simulink model "F16ASYM_Controlled_ACC"  (R2012b)
settings: Solver=ode3  SolverMode=SingleTasking  StartTime=0.0  StopTime=inf  FixedStep=T_sim  RelTol=1e-3
InitFcn:
  | load('NN_c_weights_Last_stable.mat')
values from neighbouring files (symbols this model uses):
  a1 = fitresult.p1    [Stall_protection.m]
  alpha_map_eval = ones(size(M_eval))*NaN    [Auto_trim_aid.m]    (also in Autotrim_maps.mat = [nan nan 0.277598136245 0.119432432992 0.0579479097061 0.027)
  beta_map_eval = ones(size(M_eval))*NaN    [Auto_trim_aid.m]    (also in Autotrim_maps.mat = [nan nan -0.00151549403324 0.00117807579006 -0.0052086799721)
  C_L_0 = fitresult.p2    [Stall_protection.m]
  G_eval = NaN*ones(size(M_sq,2),size(H_sq,2))    [Stall_protection.m]
  H_sq = unique(sort(H_sq))    [Stall_protection.m]
  H_sq_autotrim = min( F_envelope.H_1g):2000:max(F_envelope.H_1g)    [Auto_trim_aid.m]    (also in Autotrim_maps.mat = [0 2000 4000 6000 8000 10000 12000 14000 16000 18000])
  K_b_ACC = params(3)    [Cost_function.m]
  K_b_q = params(4)    [Cost_function.m]
  learning = 20    [Scheduling_desing.m]
  M_sq = unique(sort(M_sq))    [Stall_protection.m]
  M_sq_autotrim = 0:0.1:max(F_envelope.M_1g)    [Auto_trim_aid.m]    (also in Autotrim_maps.mat = [0 0.1 0.2 0.3 0.4 0.5 0.6 0.7 0.8 0.9 1 1.1 ... (21 element)
  Model_used_flag = 1    [Scheduling_desing.m]
  reg_param = 1    [Scheduling_desing.m]
  T_sim = 0.04    [Run_me.m]    (also in Scheduling_desing.m = 0.02)
  tau_ACC = params(1)    [Cost_function.m]
  tau_q = params(2)    [Cost_function.m]
  V_Comp_A_w_z_last = [-0.043311742939 0.0085685727899 -0.0213735657625 0.0330213821126 -0.0306555996667 -0.00573122365227 -0.0106441480787 0.0329440631876 0.0177121952361 -0.0290685435098 -0.0181457235686 -0.0361990502411 ... (1250 elements, 50x25)]    [NN_c_weights_Last_stable.mat]
  V_Comp_last = [-0.0421958473648 0.0184516098779 -0.0436695953504 -0.041154016657 0.00216882652165 -0.0388561228631 0.0327521861474 0.0326079628857 0.0227071838361 -0.0338588476214 0.0161615063846 0.00186003522421 ... (1250 elements, 50x25)]    [NN_c_weights_Last_stable.mat]
  velocity = M_eval(I,J)*a    [Auto_trim_aid.m]    (also in Scheduling_desing.m = M_eval_sche(I,J)*a)
  W_Comp_A_w_z_last = [-0.00689921461652 0.00234704735165 -0.000126421245896 0.00121944724496 6.17702028018e-05 -0.000422762754226 -0.000228913732743 -1.1618795843e-05 7.94007436465e-05 0.000588815786054 2.98617078429e-05 -0.00020420127191 ... (153 elements, 3x51)]    [NN_c_weights_Last_stable.mat]
  W_Comp_last = [-0.00864477030284 0.000183920433695 -0.000300268209456 0.00178165628538 -0.000144806488148 -0.000715209966 -0.000733452792184 5.9552378004e-05 0.000293789747621 0.00184648331608 -0.000150090451416 -0.000741280397229 ... (153 elements, 3x51)]    [NN_c_weights_Last_stable.mat]
undefined symbols (not defined in the file or in its folder): B, DiscIntNeverNeededParam, fi_flag_Simulink, k_B, m_B, sigbuilder_block, Stall_curve, Theta_1_roll_last, Theta_2_roll_last, Theta_3_roll_last, trim_control, trim_state, trim_throttle, V_long_lastA_w_z, V_long_lastAoA, V_roll_last, V_roll_lastMOD, V_yaw_last, W_long_lastA_w_z, W_long_lastAoA, W_roll_last, W_roll_lastMOD, W_yaw_last
libraries: Adaptive_FaultTolerantControl x43, F16_Actuator_Library x14, dspsigops x13, simulink x8, dsparch4 x6, simulink_extras x5, aerolibatmos2 x5, aerolibtransform2 x5, dspmtrx3 x3, qcatlib x2, dspvision x2, dspsnks4 x2
(part 7 of 10)

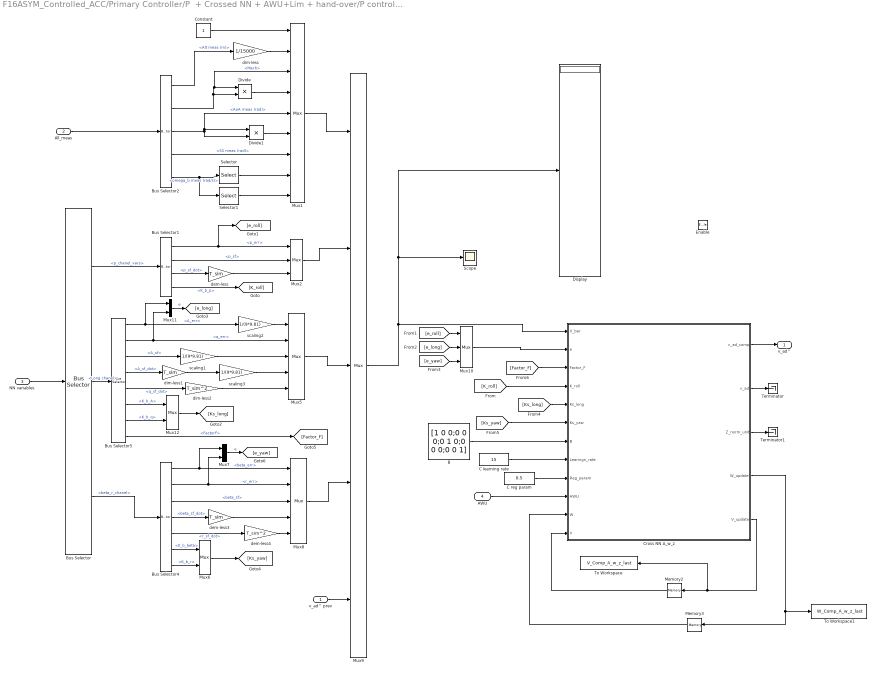
== system F16ASYM_Controlled_ACC/Primary Controller/P  + Crossed NN + AWU+Lim + hand-over/P controller + adaptive Crossed NN + AWU+Lim    in ACC /Complete crossed On-line (adaptive) multi-layer NN: A_w_z ==
  v_ad^ prev : Inport
  All_meas : Inport  Port=2
  NN variables : Inport  Port=3
  AWU : Inport  Port=4
  Enable : EnablePort  StatesWhenEnabling=reset
  B : Constant  Value=[1 0 0;0 0 0;0 1 0;0 0 0;0 0 1]
  Bus Selector : BusSelector  OutputSignals=p_chanel_vars,Long chanel,beta_r_chanel
  Bus Selector1 : BusSelector  OutputSignals=p_err,p_sf,p_sf_dot,K_b_p
  Bus Selector2 : BusSelector  OutputSignals=signal1.Alt meas (m),signal2.Mach,signal1.AoA meas (rad),signal1.SS meas (rad),signal1.omega_b meas (rad/s)
  Bus Selector4 : BusSelector  OutputSignals=beta_chanel vars.beta_err,r_chanel vars.r_err,beta_chanel vars.beta_sf,beta_chanel vars.beta_sf_dot,r_chanel vars.r_sf_dot,beta_chanel vars.K_b_beta,r_chanel vars.K_b_r
  Bus Selector5 : BusSelector  OutputSignals=A_chanel vars.A_err,q_chanel_vars.q_err,A_chanel vars.A_sf,A_chanel vars.A_sf_dot,q_chanel_vars.q_sf_dot,A_chanel vars.K_b_A,q_chanel_vars.K_b_q,A_chanel vars.FactorF
  C learning rate : Constant  Value=15  SampleTime=T_sim
  C reg param : Constant  Value=0.5  SampleTime=T_sim
  Constant : Constant
  Cross NN A_w_z : MATLAB Function  TreatAsAtomicUnit=on
  Display : Display
  Divide : Product  Inputs=**
  Divide1 : Product  Inputs=**
  Memory2 : Memory  X0=V_Comp_A_w_z_last
  Memory3 : Memory  X0=W_Comp_A_w_z_last
  Mux1 : Mux  Inputs=9
  Mux10 : Mux  Inputs=3
  Mux{6..7,11..12} (4 alike) : Mux  Inputs=2
  Mux2 : Mux  Inputs=3
  Mux5 : Mux  Inputs=5
  Mux8 : Mux  Inputs=5
  Mux9 : Mux  Inputs=[9 3 5 5 3]
  Scope : Scope
      settings: SaveName=ScopeData8
  Selector : Selector  InputPortWidth=3  IndexOptions=Index vector (dialog)  Indices=1  OutputSizes=1
  Selector1 : Selector  InputPortWidth=3  IndexOptions=Index vector (dialog)  Indices=3  OutputSizes=1
  Terminator : Terminator
  Terminator1 : Terminator
  To Workspace : ToWorkspace  VariableName=V_Comp_A_w_z_last  SampleTime=-1
      settings: MaxDataPoints=1
  To Workspace1 : ToWorkspace  VariableName=W_Comp_A_w_z_last  SampleTime=-1
      settings: MaxDataPoints=1
  dem-less : Gain  Gain=T_sim
  dem-less3 : Gain  Gain=T_sim
  dem-less4 : Gain  Gain=T_sim^2
  dim-less : Gain  Gain=1/15000
  dim-less1 : Gain  Gain=T_sim
  dim-less2 : Gain  Gain=T_sim^2
  scaling1 : Gain  Gain=1/(9*9.81)
  scaling2 : Gain  Gain=1/(9*9.81)
  scaling3 : Gain  Gain=1/(9*9.81)
  v_ad^ : Outport
  wires:
  [Factor_F] -> Cross NN A_w_z/3(Factor_F)
  Bus Selector5/8 -> [Factor_F]  "<FactorF>"
  scaling3/1 -> Mux5/4
  dim-less2/1 -> Mux5/5
  scaling1/1 -> Mux5/3
  Mux11/1 -> [e_long]  "e"
  Bus Selector/2 -> Bus Selector5/1  "<Long chanel>"
  Bus Selector5/1 -> Mux11/1, scaling2/1  "<A_err>"
  Bus Selector5/2 -> Mux11/2, Mux5/2  "<q_err>"
  Bus Selector5/3 -> scaling1/1  "<A_sf>"
  Bus Selector5/4 -> dim-less1/1  "<A_sf_dot>"
  Bus Selector5/5 -> dim-less2/1  "<q_sf_dot>"
  Bus Selector5/7 -> Mux12/2  "<K_b_q>"
  Bus Selector5/6 -> Mux12/1  "<K_b_A>"
  scaling2/1 -> Mux5/1
  dim-less1/1 -> scaling3/1
  Selector1/1 -> Mux1/9
  [Ks_yaw] -> Cross NN A_w_z/6(Ks_yaw)
  [Ks_long] -> Cross NN A_w_z/5(Ks_long)
  [K_roll] -> Cross NN A_w_z/4(K_roll)
  [e_yaw] -> Mux10/3
  [e_long] -> Mux10/2
  [e_roll] -> Mux10/1
  Mux10/1 -> Cross NN A_w_z/2(e)
  Cross NN A_w_z/4(W_update) -> To Workspace1/1, Memory3/1
  Cross NN A_w_z/5(V_update) -> Memory2/1, To Workspace/1
  Cross NN A_w_z/2(v_ad) -> Terminator/1
  B/1 -> Cross NN A_w_z/7(B)
  Memory3/1 -> Cross NN A_w_z/11(W)
  Memory2/1 -> Cross NN A_w_z/12(V)
  Cross NN A_w_z/1(v_ad_comp) -> v_ad^/1
  C learning rate/1 -> Cross NN A_w_z/8(Learnign_rate)
  C reg param/1 -> Cross NN A_w_z/9(Reg_param)
  Cross NN A_w_z/3(Z_norm_unit) -> Terminator1/1
  Mux9/1 -> Cross NN A_w_z/1(X_bar), Display/1, Scope/1
  v_ad^ prev/1 -> Mux9/5
  Mux8/1 -> Mux9/4
  Mux5/1 -> Mux9/3
  Mux2/1 -> Mux9/2
  Mux1/1 -> Mux9/1
  dem-less4/1 -> Mux8/5
  Mux7/1 -> [e_yaw]  "e"
  Bus Selector4/2 -> Mux7/2, Mux8/2  "<r_err>"
  Bus Selector4/1 -> Mux7/1, Mux8/1  "<beta_err>"
  Mux6/1 -> [Ks_yaw]
  Bus Selector4/6 -> Mux6/1  "<K_b_beta>"
  Bus Selector4/7 -> Mux6/2  "<K_b_r>"
  Bus Selector4/5 -> dem-less4/1  "<r_sf_dot>"
  Bus Selector4/4 -> dem-less3/1  "<beta_sf_dot>"
  Bus Selector4/3 -> Mux8/3  "<beta_sf>"
  dem-less3/1 -> Mux8/4
  Mux12/1 -> [Ks_long]
  dem-less/1 -> Mux2/3
  Bus Selector1/1 -> Mux2/1, [e_roll]  "<p_err>"
  Bus Selector1/2 -> Mux2/2  "<p_sf>"
  Bus Selector1/4 -> [K_roll]  "<K_b_p>"
  Bus Selector2/3 -> Divide1/2, Mux1/5, Divide1/1  "<AoA meas (rad)>"
  Bus Selector2/2 -> Divide/1, Mux1/3, Divide/2  "<Mach>"
  Bus Selector2/4 -> Mux1/7  "<SS meas (rad)>"
  Selector/1 -> Mux1/8
  Bus Selector1/3 -> dem-less/1  "<p_sf_dot>"
  Constant/1 -> Mux1/1
  All_meas/1 -> Bus Selector2/1
  Bus Selector2/1 -> dim-less/1  "<Alt meas (m)>"
  Divide/1 -> Mux1/4
  Divide1/1 -> Mux1/6
  dim-less/1 -> Mux1/2
  Bus Selector2/5 -> Selector/1, Selector1/1  "<omega_b meas (rad/s)>"
  NN variables/1 -> Bus Selector/1
  Bus Selector/1 -> Bus Selector1/1  "<p_chanel_vars>"
  Bus Selector/3 -> Bus Selector4/1  "<beta_r_chanel>"
  AWU/1 -> Cross NN A_w_z/10(AWU)

== system F16ASYM_Controlled_ACC/Primary Controller/P  + Crossed NN + AWU+Lim + hand-over/P controller + adaptive Crossed NN + AWU+Lim    in ACC /Lat_dir Dyn Inversion: beta_dot->r_c ==
  beta_dot_c : Inport
  All_meas : Inport  Port=2
  A_w_y : Selector  InputPortWidth=3  IndexOptions=Index vector (dialog)  Indices=2  OutputSizes=1
  Bus Selector : BusSelector  OutputSignals=signal1.AoA meas (rad),signal1.omega_b meas (rad/s),signal1.V_TAS (m/s),signal2.A_w_CG
  Divide1 : Product  Inputs=**
  Divide3 : Product  Inputs=**
  Divide4 : Product  Inputs=/*
  Divide5 : Product  Inputs=*/
  Selector : Selector  InputPortWidth=3  IndexOptions=Index vector (dialog)  Indices=1  OutputSizes=1
  Trigonometric Function : Trigonometry  Operator=cos
  Trigonometric Function3 : Trigonometry  Operator=tan
  "q_c " : Sum  Inputs=-++
  r_c : Outport
  wires:
  "q_c "/1 -> r_c/1
  Bus Selector/1 -> Trigonometric Function/1, Trigonometric Function3/1  "<AoA meas (rad)>"
  Bus Selector/2 -> Selector/1  "<omega_b meas (rad/s)>"
  Divide1/1 -> "q_c "/2
  Divide3/1 -> Divide4/1
  A_w_y/1 -> Divide4/2
  All_meas/1 -> Bus Selector/1
  Bus Selector/4 -> A_w_y/1  "<A_w_CG>"
  Divide4/1 -> "q_c "/3
  Bus Selector/3 -> Divide3/2  "<V_TAS (m/s)>"
  Trigonometric Function/1 -> Divide3/1, Divide5/2
  Divide5/1 -> "q_c "/1
  beta_dot_c/1 -> Divide5/1
  Trigonometric Function3/1 -> Divide1/1
  Selector/1 -> Divide1/2

== system F16ASYM_Controlled_ACC/Primary Controller/P  + Crossed NN + AWU+Lim + hand-over/P controller + adaptive Crossed NN + AWU+Lim    in ACC /Long Dyn Inversion: alpha_dot ->q ==
  alpha_dot_c : Inport
  All_meas : Inport  Port=2
  Completed : Subsystem
  Manual Switch : ManualSwitch
  Simplified : Subsystem
  q_c : Outport
  wires:
  alpha_dot_c/1 -> Simplified/1(alpha_dot_c), Completed/1(alpha_dot_c)
  All_meas/1 -> Simplified/2(All_meas), Completed/2(All_meas)
  Completed/1(q_c) -> Manual Switch/1
  Simplified/1(q_c) -> Manual Switch/2
  Manual Switch/1 -> q_c/1

== system F16ASYM_Controlled_ACC/Primary Controller/P  + Crossed NN + AWU+Lim + hand-over/P controller + adaptive Crossed NN + AWU+Lim    in ACC /Longitudinal controller in A_w_z ==
  A_w_z des : Inport
  AoA des (rad) : Inport  Port=2
  Anti-windup A_w_z : Inport  Port=3
  Anti-windup AoA : Inport  Port=4
  All meas : Inport  Port=5
  Accel rate --> AoA rate! : Subsystem
  Bus Creator : BusCreator  Inputs=5
  Bus Selector : BusSelector  OutputSignals=signal2.A_w_CG
  Divide : Product  Inputs=**
  Gain : Gain  Gain=-1
  Ref Model and P Controller : Adaptive_FaultTolerantControl/Ref Model and P Controller  tau=0.3  y_i=0  K_f=1  K_b=2.5
  Selector : Selector  InputPortWidth=3  IndexOptions=Index vector (dialog)  Indices=3  OutputSizes=1
  Stall protection : Subsystem  Commented=on
  Sum : Sum  Inputs=+-|
  Terminator : Terminator
  Terminator1 : Terminator
  Terminator2 : Terminator
  A_chanel vars : Outport
  alpha_dot_c : Outport  Port=2
  wires:
  Anti-windup AoA/1 -> Terminator1/1
  AoA des (rad)/1 -> Terminator/1
  Selector/1 -> Gain/1
  Gain/1 -> Ref Model and P Controller/2
  Bus Selector/1 -> Selector/1  "<A_w_CG>"
  Anti-windup A_w_z/1 -> Terminator2/1
  A_w_z des/1 -> Ref Model and P Controller/1
  Ref Model and P Controller/1 -> Divide/1
  Ref Model and P Controller/2 -> Bus Creator/1  "A_sf_dot"
  Ref Model and P Controller/3 -> Bus Creator/2, Sum/1  "A_sf"
  Sum/1 -> Bus Creator/3  "A_err"
  Ref Model and P Controller/4 -> Sum/2
  Ref Model and P Controller/5 -> Bus Creator/4  "K_b_A"
  Bus Creator/1 -> A_chanel vars/1
  Divide/1 -> alpha_dot_c/1
  Accel rate --> AoA rate!/1(A_w  to AoA rates factor) -> Bus Creator/5, Divide/2  "FactorF"
  All meas/1 -> Bus Selector/1, Stall protection/2(All meas), Accel rate --> AoA rate!/1(All_meas)

== system F16ASYM_Controlled_ACC/Primary Controller/P  + Crossed NN + AWU+Lim + hand-over/P controller + adaptive Crossed NN + AWU+Lim    in ACC /Physical limitation ==
  note: Converto to Angular accelerations
  v comm : Inport
  all meas : Inport  Port=2
  Ang Accel : MATLAB Function
  Bus Selector : BusSelector  OutputSignals=signal1.Alt meas (m),signal1.V_TAS (m/s),signal1.AoA meas (rad),signal1.SS meas (rad),signal1.omega_b meas (rad/s),signal1.Throttle_meas
  Bus Selector1 : BusSelector  OutputSignals=signal2.q (Pa),signal1.omega_b meas (rad/s)
  Demux : Demux  Outputs=3
  Display : Display
  Display1 : Display
  Display2 : Display
  Divide : Product  Inputs=**
  Divide1 : Product  Inputs=**
  Gain : Gain  Gain=-1
  Gain1 : Gain
  Mom coefficients that was reached : MATLABFcn  MATLABFcn=Moms_Coeff_estimator  OutputDimensions=3  OutputSignalType=real
  Moments : Subsystem
  Mux : Mux  Inputs=3
  Mux1 : Mux  Inputs=7
  Saturation Dynamic : simulink/Discontinuities/Saturation Dynamic  OutMin=[]  OutMax=[]  OutDataTypeStr=Inherit: Same as second input  OutDataType=fixdt(1, 16)  OutScaling=2^-10  DoSatur=off
  Sign : Signum
  Sign1 : Signum
  max deflections estimator : MATLAB Function  TreatAsAtomicUnit=on
  v limted : Outport
  wires:
  max deflections estimator/1(max_defl) -> Mux1/7
  Mux1/1 -> Mom coefficients that was reached/1
  Bus Selector/5 -> Mux1/5  "<omega_b meas (rad/s)>"
  Bus Selector/1 -> Mux1/1  "<Alt meas (m)>"
  Bus Selector/2 -> Mux1/2  "<V_TAS (m/s)>"
  Bus Selector/3 -> Mux1/3  "<AoA meas (rad)>"
  Bus Selector/4 -> Mux1/4  "<SS meas (rad)>"
  Bus Selector/6 -> Mux1/6  "<Throttle_meas>"
  Ang Accel/2(q_dot) -> Mux/2
  Ang Accel/3(r_dot) -> Mux/3
  Ang Accel/1(p_dot) -> Mux/1
  Bus Selector1/2 -> Ang Accel/4(omega_b)  "<omega_b meas (rad/s)>"
  Moments/3(N) -> Ang Accel/3(N)
  Moments/2(M) -> Ang Accel/2(M)
  Moments/1(L) -> Ang Accel/1(L)
  Bus Selector1/1 -> Moments/4(q)  "<q (Pa)>"
  Demux/3 -> Moments/3(C_N)
  Demux/2 -> Moments/2(C_M)
  Demux/1 -> Moments/1(C_L)
  Mom coefficients that was reached/1 -> Demux/1
  all meas/1 -> Bus Selector/1, Bus Selector1/1
  Mux/1 -> Gain1/1
  v comm/1 -> Saturation Dynamic/2, Display1/1, max deflections estimator/1(v_comm)
  Saturation Dynamic/1 -> Display/1, v limted/1
  Sign/1 -> Divide/1
  Gain1/1 -> Divide/2, Divide1/1, Sign1/1, Display2/1, Sign/1
  Sign1/1 -> Gain/1
  Divide/1 -> Saturation Dynamic/1
  Gain/1 -> Divide1/2
  Divide1/1 -> Saturation Dynamic/3

== system F16ASYM_Controlled_ACC/Primary Controller/P  + Crossed NN + AWU+Lim + hand-over/P controller + adaptive Crossed NN + AWU+Lim    in ACC /Sigmoid  ==
  In : Inport
  Display : Display
  Fcn1 : Fcn  Commented=on  Expr=2.0 ./ (1.0 + exp(-u(4)*u(1:3)))-1
  MATLAB Function : MATLAB Function  TreatAsAtomicUnit=on
  a : Constant  Value=a
  Out : Outport
  wires:
  MATLAB Function/1(y) -> Display/1, Out/1
  In/1 -> MATLAB Function/1(u)
  a/1 -> MATLAB Function/2(a)

== system F16ASYM_Controlled_ACC/Primary Controller/P  + Crossed NN + AWU+Lim + hand-over/P controller + adaptive Crossed NN + AWU+Lim   in AoA/Body Rates Controller ==
  p_ref : Inport
  q_ref : Inport  Port=2
  r_ref : Inport  Port=3
  All_meas : Inport  Port=4
  Bus Creator : BusCreator
  Bus Creator1 : BusCreator
  Bus Creator2 : BusCreator
  Bus Selector : BusSelector  OutputSignals=signal1.omega_b meas (rad/s)
  Display1 : Display
  Mux : Mux  Inputs=3
  Ref Model and P Controller p : Adaptive_FaultTolerantControl/Ref Model and P Controller  tau=0.1  y_i=trim_state(10)  K_f=1  K_b=7
  Ref Model and P Controller q : Adaptive_FaultTolerantControl/Ref Model and P Controller  tau=0.06  y_i=trim_state(11)  K_f=1  K_b=1
  Ref Model and P Controller r : Adaptive_FaultTolerantControl/Ref Model and P Controller  tau=0.2  y_i=trim_state(12)  K_f=1  K_b=4
  Selector : Selector  InputPortWidth=3  IndexOptions=Index vector (dialog)  Indices=1  OutputSizes=1
  Selector1 : Selector  InputPortWidth=3  IndexOptions=Index vector (dialog)  Indices=2  OutputSizes=1
  Selector2 : Selector  InputPortWidth=3  IndexOptions=Index vector (dialog)  Indices=3  OutputSizes=1
  Sum : Sum  Inputs=+-|
  Sum1 : Sum  Inputs=+-|
  Sum2 : Sum  Inputs=+-|
  q_chanel vars : Outport
  p_chanel vars : Outport  Port=2
  r_chanel vars : Outport  Port=3
  Angular acc des (rad/s^2) : Outport  Port=4
  wires:
  All_meas/1 -> Bus Selector/1
  Bus Selector/1 -> Selector/1, Selector1/1, Selector2/1  "<omega_b meas (rad/s)>"
  p_ref/1 -> Ref Model and P Controller p/1
  Selector/1 -> Ref Model and P Controller p/2
  Ref Model and P Controller p/1 -> Mux/1
  Mux/1 -> Angular acc des (rad/s^2)/1
  q_ref/1 -> Ref Model and P Controller q/1
  Selector1/1 -> Ref Model and P Controller q/2
  r_ref/1 -> Ref Model and P Controller r/1
  Ref Model and P Controller q/1 -> Mux/2
  Ref Model and P Controller r/1 -> Mux/3
  Ref Model and P Controller p/2 -> Bus Creator/1  "p_sf_dot"
  Ref Model and P Controller p/3 -> Sum/1, Bus Creator/2  "p_sf"
  Sum/1 -> Display1/1, Bus Creator/3  "p_err"
  Bus Creator/1 -> p_chanel vars/1
  Bus Creator1/1 -> q_chanel vars/1
  Bus Creator2/1 -> r_chanel vars/1
  Selector2/1 -> Ref Model and P Controller r/2
  Ref Model and P Controller p/4 -> Sum/2
  Ref Model and P Controller p/5 -> Bus Creator/4  "K_b_p"
  Ref Model and P Controller q/2 -> Bus Creator1/1  "q_sf_dot"
  Ref Model and P Controller q/3 -> Sum1/1, Bus Creator1/2  "q_sf"
  Sum1/1 -> Bus Creator1/3  "q_err"
  Ref Model and P Controller q/4 -> Sum1/2
  Ref Model and P Controller q/5 -> Bus Creator1/4  "K_b_q"
  Ref Model and P Controller r/2 -> Bus Creator2/1  "r_sf_dot"
  Ref Model and P Controller r/3 -> Sum2/1, Bus Creator2/2  "r_sf"
  Sum2/1 -> Bus Creator2/3  "r_err"
  Ref Model and P Controller r/4 -> Sum2/2
  Ref Model and P Controller r/5 -> Bus Creator2/4  "K_b_r"

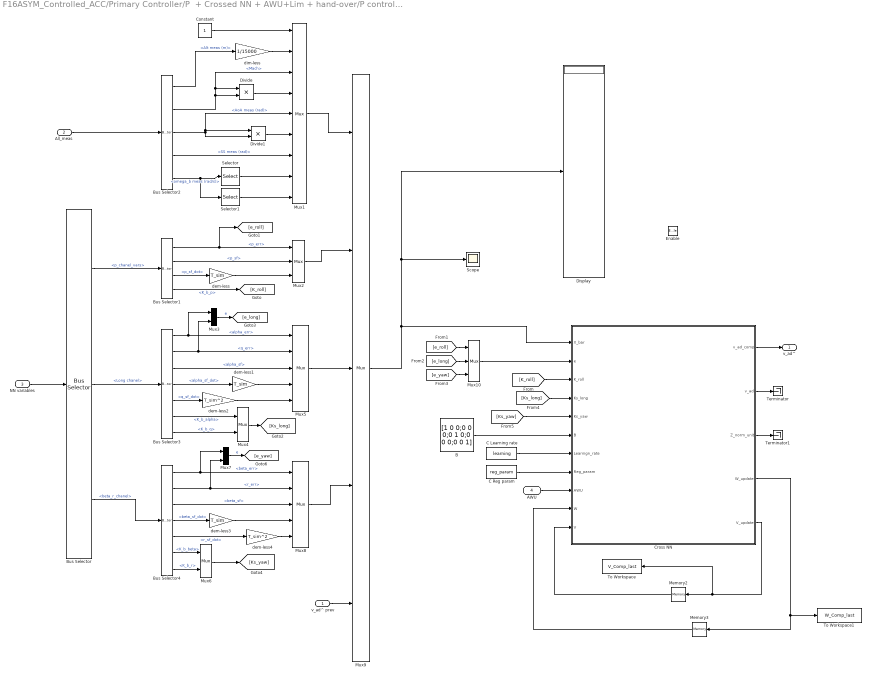
== system F16ASYM_Controlled_ACC/Primary Controller/P  + Crossed NN + AWU+Lim + hand-over/P controller + adaptive Crossed NN + AWU+Lim   in AoA/Complete crossed On-line (adaptive) multi-layer NN: AoA ==
  v_ad^ prev : Inport
  All_meas : Inport  Port=2
  NN variables : Inport  Port=3
  AWU : Inport  Port=4
  Enable : EnablePort  StatesWhenEnabling=reset
  B : Constant  Value=[1 0 0;0 0 0;0 1 0;0 0 0;0 0 1]
  Bus Selector : BusSelector  OutputSignals=p_chanel_vars,Long chanel,beta_r_chanel
  Bus Selector1 : BusSelector  OutputSignals=p_err,p_sf,p_sf_dot,K_b_p
  Bus Selector2 : BusSelector  OutputSignals=signal1.Alt meas (m),signal2.Mach,signal1.AoA meas (rad),signal1.SS meas (rad),signal1.omega_b meas (rad/s)
  Bus Selector3 : BusSelector  OutputSignals=alpha_chanel vars.alpha_err,q_chanel_vars.q_err,alpha_chanel vars.alpha_sf,alpha_chanel vars.alpha_sf_dot,q_chanel_vars.q_sf_dot,alpha_chanel vars.K_b_alpha,q_chanel_vars.K_b_q
  Bus Selector4 : BusSelector  OutputSignals=beta_chanel vars.beta_err,r_chanel vars.r_err,beta_chanel vars.beta_sf,beta_chanel vars.beta_sf_dot,r_chanel vars.r_sf_dot,beta_chanel vars.K_b_beta,r_chanel vars.K_b_r
  C Learning rate : Constant  Value=learning  SampleTime=T_sim
  C Reg param : Constant  Value=reg_param  SampleTime=T_sim
  Constant : Constant
  Cross NN : MATLAB Function  TreatAsAtomicUnit=on
  Display : Display
  Divide : Product  Inputs=**
  Divide1 : Product  Inputs=**
  Memory2 : Memory  X0=V_Comp_last
  Memory3 : Memory  X0=W_Comp_last
  Mux1 : Mux  Inputs=9
  Mux10 : Mux  Inputs=3
  Mux2 : Mux  Inputs=3
  Mux{3..4,6..7} (4 alike) : Mux  Inputs=2
  Mux5 : Mux  Inputs=5
  Mux8 : Mux  Inputs=5
  Mux9 : Mux  Inputs=[9 3 5 5 3]
  Scope : Scope
      settings: SaveName=ScopeData8
  Selector : Selector  InputPortWidth=3  IndexOptions=Index vector (dialog)  Indices=1  OutputSizes=1
  Selector1 : Selector  InputPortWidth=3  IndexOptions=Index vector (dialog)  Indices=3  OutputSizes=1
  Terminator : Terminator
  Terminator1 : Terminator
  To Workspace : ToWorkspace  VariableName=V_Comp_last  SampleTime=-1
      settings: MaxDataPoints=1
  To Workspace1 : ToWorkspace  VariableName=W_Comp_last  SampleTime=-1
      settings: MaxDataPoints=1
  dem-less : Gain  Gain=T_sim
  dem-less1 : Gain  Gain=T_sim
  dem-less2 : Gain  Gain=T_sim^2
  dem-less3 : Gain  Gain=T_sim
  dem-less4 : Gain  Gain=T_sim^2
  dim-less : Gain  Gain=1/15000
  v_ad^ : Outport
  wires:
  Bus Selector/3 -> Bus Selector4/1  "<beta_r_chanel>"
  Bus Selector/2 -> Bus Selector3/1  "<Long chanel>"
  Bus Selector/1 -> Bus Selector1/1  "<p_chanel_vars>"
  NN variables/1 -> Bus Selector/1
  Bus Selector2/5 -> Selector1/1, Selector/1  "<omega_b meas (rad/s)>"
  dim-less/1 -> Mux1/2
  Divide1/1 -> Mux1/6
  Divide/1 -> Mux1/4
  Bus Selector2/1 -> dim-less/1  "<Alt meas (m)>"
  All_meas/1 -> Bus Selector2/1
  Constant/1 -> Mux1/1
  Bus Selector1/3 -> dem-less/1  "<p_sf_dot>"
  Selector/1 -> Mux1/8
  Bus Selector2/4 -> Mux1/7  "<SS meas (rad)>"
  Bus Selector2/2 -> Divide/2, Mux1/3, Divide/1  "<Mach>"
  Bus Selector2/3 -> Divide1/1, Mux1/5, Divide1/2  "<AoA meas (rad)>"
  Bus Selector1/4 -> [K_roll]  "<K_b_p>"
  Bus Selector1/2 -> Mux2/2  "<p_sf>"
  Bus Selector1/1 -> [e_roll], Mux2/1  "<p_err>"
  dem-less/1 -> Mux2/3
  dem-less2/1 -> Mux5/5
  dem-less1/1 -> Mux5/4
  Mux4/1 -> [Ks_long]
  Bus Selector3/6 -> Mux4/1  "<K_b_alpha>"
  Bus Selector3/7 -> Mux4/2  "<K_b_q>"
  Bus Selector3/5 -> dem-less2/1  "<q_sf_dot>"
  Bus Selector3/4 -> dem-less1/1  "<alpha_sf_dot>"
  Bus Selector3/1 -> Mux5/1, Mux3/1  "<alpha_err>"
  Bus Selector3/2 -> Mux5/2, Mux3/2  "<q_err>"
  Bus Selector3/3 -> Mux5/3  "<alpha_sf>"
  Mux3/1 -> [e_long]  "e"
  dem-less3/1 -> Mux8/4
  Bus Selector4/3 -> Mux8/3  "<beta_sf>"
  Bus Selector4/4 -> dem-less3/1  "<beta_sf_dot>"
  Bus Selector4/5 -> dem-less4/1  "<r_sf_dot>"
  Bus Selector4/7 -> Mux6/2  "<K_b_r>"
  Bus Selector4/6 -> Mux6/1  "<K_b_beta>"
  Mux6/1 -> [Ks_yaw]
  Bus Selector4/1 -> Mux8/1, Mux7/1  "<beta_err>"
  Bus Selector4/2 -> Mux8/2, Mux7/2  "<r_err>"
  Mux7/1 -> [e_yaw]  "e"
  dem-less4/1 -> Mux8/5
  Mux1/1 -> Mux9/1
  Mux2/1 -> Mux9/2
  Mux5/1 -> Mux9/3
  Mux8/1 -> Mux9/4
  v_ad^ prev/1 -> Mux9/5
  Mux9/1 -> Scope/1, Display/1, Cross NN/1(X_bar)
  Cross NN/3(Z_norm_unit) -> Terminator1/1
  C Reg param/1 -> Cross NN/8(Reg_param)
  C Learning rate/1 -> Cross NN/7(Learnign_rate)
  Cross NN/1(v_ad_comp) -> v_ad^/1
  Memory2/1 -> Cross NN/11(V)
  Memory3/1 -> Cross NN/10(W)
  B/1 -> Cross NN/6(B)
  Cross NN/2(v_ad) -> Terminator/1
  Cross NN/5(V_update) -> To Workspace/1, Memory2/1
  Cross NN/4(W_update) -> Memory3/1, To Workspace1/1
  Mux10/1 -> Cross NN/2(e)
  [e_roll] -> Mux10/1
  [e_long] -> Mux10/2
  [e_yaw] -> Mux10/3
  [K_roll] -> Cross NN/3(K_roll)
  [Ks_long] -> Cross NN/4(Ks_long)
  [Ks_yaw] -> Cross NN/5(Ks_yaw)
  Selector1/1 -> Mux1/9
  AWU/1 -> Cross NN/9(AWU)

== system F16ASYM_Controlled_ACC/Primary Controller/P  + Crossed NN + AWU+Lim + hand-over/P controller + adaptive Crossed NN + AWU+Lim   in AoA/Lat_dir Dyn Inversion: beta_dot->r_c ==
  beta_dot_c : Inport
  All_meas : Inport  Port=2
  A_w_y : Selector  InputPortWidth=3  IndexOptions=Index vector (dialog)  Indices=2  OutputSizes=1
  Bus Selector : BusSelector  OutputSignals=signal1.AoA meas (rad),signal1.omega_b meas (rad/s),signal1.V_TAS (m/s),signal2.A_w_CG
  Divide1 : Product  Inputs=**
  Divide3 : Product  Inputs=**
  Divide4 : Product  Inputs=/*
  Divide5 : Product  Inputs=*/
  Selector : Selector  InputPortWidth=3  IndexOptions=Index vector (dialog)  Indices=1  OutputSizes=1
  Trigonometric Function : Trigonometry  Operator=cos
  Trigonometric Function3 : Trigonometry  Operator=tan
  "q_c " : Sum  Inputs=-++
  r_c : Outport
  wires:
  "q_c "/1 -> r_c/1
  Bus Selector/1 -> Trigonometric Function/1, Trigonometric Function3/1  "<AoA meas (rad)>"
  Bus Selector/2 -> Selector/1  "<omega_b meas (rad/s)>"
  Divide1/1 -> "q_c "/2
  Divide3/1 -> Divide4/1
  A_w_y/1 -> Divide4/2
  All_meas/1 -> Bus Selector/1
  Bus Selector/4 -> A_w_y/1  "<A_w_CG>"
  Divide4/1 -> "q_c "/3
  Bus Selector/3 -> Divide3/2  "<V_TAS (m/s)>"
  Trigonometric Function/1 -> Divide3/1, Divide5/2
  Divide5/1 -> "q_c "/1
  beta_dot_c/1 -> Divide5/1
  Trigonometric Function3/1 -> Divide1/1
  Selector/1 -> Divide1/2

== system F16ASYM_Controlled_ACC/Primary Controller/P  + Crossed NN + AWU+Lim + hand-over/P controller + adaptive Crossed NN + AWU+Lim   in AoA/Long Dyn Inversion: alpha_dot ->q ==
  alpha_dot_c : Inport
  All_meas : Inport  Port=2
  Completed : Subsystem
  Manual Switch : ManualSwitch
  Simplified : Subsystem
  q_c : Outport
  wires:
  alpha_dot_c/1 -> Simplified/1(alpha_dot_c), Completed/1(alpha_dot_c)
  All_meas/1 -> Simplified/2(All_meas), Completed/2(All_meas)
  Completed/1(q_c) -> Manual Switch/1
  Simplified/1(q_c) -> Manual Switch/2
  Manual Switch/1 -> q_c/1

== system F16ASYM_Controlled_ACC/Primary Controller/P  + Crossed NN + AWU+Lim + hand-over/P controller + adaptive Crossed NN + AWU+Lim   in AoA/Longitudinal controller in AoA ==
  A_w_z des : Inport
  AoA des (rad) : Inport  Port=2
  Anti-windup A_w_z : Inport  Port=3
  Anti-windup AoA : Inport  Port=4
  All meas : Inport  Port=5
  Bus Creator : BusCreator
  Bus Selector : BusSelector  OutputSignals=signal1.AoA meas (rad)
  Ref Model and P Controller : Adaptive_FaultTolerantControl/Ref Model and P Controller  tau=0.9  y_i=trim_state(8)  K_f=1  K_b=10
  Sum : Sum  Inputs=+-|
  Terminator : Terminator
  Terminator1 : Terminator
  Terminator2 : Terminator
  alpha_chanel vars : Outport
  alpha_dot_c : Outport  Port=2
  wires:
  All meas/1 -> Bus Selector/1
  Ref Model and P Controller/1 -> alpha_dot_c/1
  Bus Selector/1 -> Ref Model and P Controller/2  "<AoA meas (rad)>"
  AoA des (rad)/1 -> Ref Model and P Controller/1
  A_w_z des/1 -> Terminator/1
  Anti-windup A_w_z/1 -> Terminator1/1
  Anti-windup AoA/1 -> Terminator2/1
  Ref Model and P Controller/2 -> Bus Creator/1  "alpha_sf_dot"
  Ref Model and P Controller/3 -> Sum/1, Bus Creator/2  "alpha_sf"
  Sum/1 -> Bus Creator/3  "alpha_err"
  Bus Creator/1 -> alpha_chanel vars/1
  Ref Model and P Controller/4 -> Sum/2
  Ref Model and P Controller/5 -> Bus Creator/4  "K_b_alpha"

== system F16ASYM_Controlled_ACC/Primary Controller/P  + Crossed NN + AWU+Lim + hand-over/P controller + adaptive Crossed NN + AWU+Lim   in AoA/Physical limitation ==
  note: Converto to Angular accelerations
  v comm : Inport
  all meas : Inport  Port=2
  Ang Accel : MATLAB Function
  Bus Selector : BusSelector  OutputSignals=signal1.Alt meas (m),signal1.V_TAS (m/s),signal1.AoA meas (rad),signal1.SS meas (rad),signal1.omega_b meas (rad/s),signal1.Throttle_meas
  Bus Selector1 : BusSelector  OutputSignals=signal2.q (Pa),signal1.omega_b meas (rad/s)
  Demux : Demux  Outputs=3
  Display : Display
  Display1 : Display
  Display2 : Display
  Divide : Product  Inputs=**
  Divide1 : Product  Inputs=**
  Gain : Gain  Gain=-1
  Gain1 : Gain
  Mom coefficients that was reached : MATLABFcn  MATLABFcn=Moms_Coeff_estimator  OutputDimensions=3  OutputSignalType=real
  Moments : Subsystem
  Mux : Mux  Inputs=3
  Mux1 : Mux  Inputs=7
  Saturation Dynamic : simulink/Discontinuities/Saturation Dynamic  OutMin=[]  OutMax=[]  OutDataTypeStr=Inherit: Same as second input  OutDataType=fixdt(1, 16)  OutScaling=2^-10  DoSatur=off
  Sign : Signum
  Sign1 : Signum
  max deflections estimator : MATLAB Function  TreatAsAtomicUnit=on
  v limted : Outport
  wires:
  max deflections estimator/1(max_defl) -> Mux1/7
  Mux1/1 -> Mom coefficients that was reached/1
  Bus Selector/5 -> Mux1/5  "<omega_b meas (rad/s)>"
  Bus Selector/1 -> Mux1/1  "<Alt meas (m)>"
  Bus Selector/2 -> Mux1/2  "<V_TAS (m/s)>"
  Bus Selector/3 -> Mux1/3  "<AoA meas (rad)>"
  Bus Selector/4 -> Mux1/4  "<SS meas (rad)>"
  Bus Selector/6 -> Mux1/6  "<Throttle_meas>"
  Ang Accel/2(q_dot) -> Mux/2
  Ang Accel/3(r_dot) -> Mux/3
  Ang Accel/1(p_dot) -> Mux/1
  Bus Selector1/2 -> Ang Accel/4(omega_b)  "<omega_b meas (rad/s)>"
  Moments/3(N) -> Ang Accel/3(N)
  Moments/2(M) -> Ang Accel/2(M)
  Moments/1(L) -> Ang Accel/1(L)
  Bus Selector1/1 -> Moments/4(q)  "<q (Pa)>"
  Demux/3 -> Moments/3(C_N)
  Demux/2 -> Moments/2(C_M)
  Demux/1 -> Moments/1(C_L)
  Mom coefficients that was reached/1 -> Demux/1
  all meas/1 -> Bus Selector/1, Bus Selector1/1
  Mux/1 -> Gain1/1
  v comm/1 -> Saturation Dynamic/2, Display1/1, max deflections estimator/1(v_comm)
  Saturation Dynamic/1 -> Display/1, v limted/1
  Sign/1 -> Divide/1
  Gain1/1 -> Divide/2, Divide1/1, Sign1/1, Display2/1, Sign/1
  Sign1/1 -> Gain/1
  Divide/1 -> Saturation Dynamic/1
  Gain/1 -> Divide1/2
  Divide1/1 -> Saturation Dynamic/3

== system F16ASYM_Controlled_ACC/Primary Controller/P  + Crossed NN + AWU+Lim + hand-over/P controller + adaptive Crossed NN + AWU+Lim   in AoA/Sigmoid  ==
  In : Inport
  Display : Display
  Fcn1 : Fcn  Commented=on  Expr=2.0 ./ (1.0 + exp(-u(4)*u(1:3)))-1
  MATLAB Function : MATLAB Function  TreatAsAtomicUnit=on
  a : Constant  Value=a
  Out : Outport
  wires:
  MATLAB Function/1(y) -> Display/1, Out/1
  In/1 -> MATLAB Function/1(u)
  a/1 -> MATLAB Function/2(a)

== system F16ASYM_Controlled_ACC/Primary Controller/P  + Crossed NN + AWU+Lim + hand-over/Transitions Smotother /Timer signal ==
  Triger : Inport
  Clock : Clock
  Constant : Constant  Value=-1/time_delay
  Constant1 : Constant  Value=0
  Integrator Limited : Integrator  ExternalReset=rising  InitialCondition=1  LimitOutput=on  UpperSaturationLimit=1  LowerSaturationLimit=0
  Relational Operator : RelationalOperator  Operator=~=  OutDataTypeStr=boolean
  pusher : Switch  Threshold=time_delay+1
  Logic output : Outport
  wires:
  Constant/1 -> Integrator Limited/1
  Triger/1 -> Integrator Limited/2
  Constant1/1 -> Relational Operator/2, pusher/3
  Clock/1 -> pusher/2
  Integrator Limited/1 -> pusher/1
  pusher/1 -> Relational Operator/1
  Relational Operator/1 -> Logic output/1

== system F16ASYM_Controlled_ACC/Primary Controller/P controller/Long Dyn Inversion: alpha_dot ->q/Completed ==
  alpha_dot_c : Inport
  All_meas : Inport  Port=2
  A_w_z : Selector  InputPortWidth=3  IndexOptions=Index vector (dialog)  Indices=3  OutputSizes=1
  Add : Sum
  Bus Selector : BusSelector  OutputSignals=signal1.AoA meas (rad),signal1.omega_b meas (rad/s),signal1.SS meas (rad),signal1.V_TAS (m/s),signal2.A_w_CG
  Display : Display
  Display1 : Display
  Display2 : Display
  Divide{,1..3} (4 alike) : Product  Inputs=**
  Divide4 : Product  Inputs=/*
  Selector : Selector  InputPortWidth=3  IndexOptions=Index vector (dialog)  Indices=1  OutputSizes=1
  Selector1 : Selector  InputPortWidth=3  IndexOptions=Index vector (dialog)  Indices=3  OutputSizes=1
  Trigonometric Function : Trigonometry  Operator=sincos
  Trigonometric Function1 : Trigonometry  Operator=tan
  Trigonometric Function2 : Trigonometry  Operator=cos
  "q_c " : Sum  Inputs=++-
  q_c : Outport
  wires:
  A_w_z/1 -> Divide4/2, Display2/1
  Trigonometric Function/2 -> Divide/1
  Trigonometric Function2/1 -> Divide3/1
  Divide1/1 -> Add/2
  Trigonometric Function1/1 -> Divide2/2
  Add/1 -> Divide2/1
  Bus Selector/4 -> Divide3/2  "<V_TAS (m/s)>"
  Divide/1 -> Add/1
  "q_c "/1 -> q_c/1
  Divide4/1 -> "q_c "/3
  Bus Selector/3 -> Trigonometric Function2/1, Trigonometric Function1/1  "<SS meas (rad)>"
  Bus Selector/5 -> A_w_z/1  "<A_w_CG>"
  All_meas/1 -> Bus Selector/1
  alpha_dot_c/1 -> Display/1, "q_c "/1
  Divide3/1 -> Divide4/1
  Selector1/1 -> Divide1/2
  Divide2/1 -> Display1/1, "q_c "/2
  Bus Selector/2 -> Selector/1, Selector1/1  "<omega_b meas (rad/s)>"
  Selector/1 -> Divide/2
  Bus Selector/1 -> Trigonometric Function/1  "<AoA meas (rad)>"
  Trigonometric Function/1 -> Divide1/1

== system F16ASYM_Controlled_ACC/Primary Controller/P controller/Long Dyn Inversion: alpha_dot ->q/Simplified ==
  alpha_dot_c : Inport
  All_meas : Inport  Port=2
  A_b_z : Selector  InputPortWidth=3  IndexOptions=Index vector (dialog)  Indices=3  OutputSizes=1
  Bus Selector : BusSelector  OutputSignals=signal2.A_b_CG,signal1.V_TAS (m/s)
  Display : Display
  Divide4 : Product  Inputs=*/
  "q_c " : Sum  Inputs=+-
  q_c : Outport
  wires:
  Bus Selector/1 -> A_b_z/1  "<A_b_CG>"
  A_b_z/1 -> Divide4/1  "A_b_z"
  Divide4/1 -> "q_c "/2
  Bus Selector/2 -> Divide4/2  "<V_TAS (m/s)>"
  alpha_dot_c/1 -> Display/1, "q_c "/1
  All_meas/1 -> Bus Selector/1
  "q_c "/1 -> q_c/1

== system F16ASYM_Controlled_ACC/Primary Controller/P controller/Longitudinal Controller: AoA or A_w_z/Longitudinal controller in A_w_z ==
  A_w_z des : Inport
  AoA des (rad) : Inport  Port=2
  Anti-windup A_w_z : Inport  Port=3
  Anti-windup AoA : Inport  Port=4
  All meas : Inport  Port=5
  Accel rate --> AoA rate! : Subsystem
  Bus Creator : BusCreator
  Bus Selector : BusSelector  OutputSignals=signal2.A_w_CG
  Gain : Gain  Gain=-1
  Ground : Ground
  Ref Model and P Controller : Adaptive_FaultTolerantControl/Ref Model and P Controller  tau=0.3  y_i=0  K_f=1  K_b=2
  Selector : Selector  InputPortWidth=3  IndexOptions=Index vector (dialog)  Indices=3  OutputSizes=1
  Sum : Sum  Inputs=+-|
  Terminator : Terminator
  Terminator1 : Terminator
  Terminator2 : Terminator
  A_chanel vars : Outport
  alpha_chanel vars : Outport  Port=2
  alpha_dot_c : Outport  Port=3
  wires:
  Ground/1 -> alpha_chanel vars/1
  Bus Creator/1 -> A_chanel vars/1
  Ref Model and P Controller/5 -> Bus Creator/4  "K_b_A"
  Ref Model and P Controller/4 -> Sum/2
  Sum/1 -> Bus Creator/3  "A_err"
  Ref Model and P Controller/3 -> Sum/1, Bus Creator/2  "A_sf"
  Ref Model and P Controller/2 -> Bus Creator/1  "A_sf_dot"
  Ref Model and P Controller/1 -> Accel rate --> AoA rate!/1(A_w_z dot)
  A_w_z des/1 -> Ref Model and P Controller/1
  Anti-windup A_w_z/1 -> Terminator2/1
  All meas/1 -> Accel rate --> AoA rate!/2(All_meas), Bus Selector/1
  Bus Selector/1 -> Selector/1  "<A_w_CG>"
  Accel rate --> AoA rate!/1(alpha_dot des) -> alpha_dot_c/1
  Gain/1 -> Ref Model and P Controller/2
  Selector/1 -> Gain/1
  AoA des (rad)/1 -> Terminator/1
  Anti-windup AoA/1 -> Terminator1/1

== system F16ASYM_Controlled_ACC/Primary Controller/P controller/Longitudinal Controller: AoA or A_w_z/Longitudinal controller in AoA ==
  A_w_z des : Inport
  AoA des (rad) : Inport  Port=2
  Anti-windup A_w_z : Inport  Port=3
  Anti-windup AoA : Inport  Port=4
  All meas : Inport  Port=5
  Bus Creator : BusCreator
  Bus Selector : BusSelector  OutputSignals=signal1.AoA meas (rad)
  Ground : Ground
  Ref Model and P Controller : Adaptive_FaultTolerantControl/Ref Model and P Controller  tau=0.8  y_i=trim_state(8)  K_f=1  K_b=10
  Sum : Sum  Inputs=+-|
  Terminator : Terminator
  Terminator1 : Terminator
  Terminator2 : Terminator
  A_chanel vars : Outport
  alpha_chanel vars : Outport  Port=2
  alpha_dot_c : Outport  Port=3
  wires:
  Ground/1 -> A_chanel vars/1
  Ref Model and P Controller/5 -> Bus Creator/4  "K_b_alpha"
  Ref Model and P Controller/4 -> Sum/2
  Bus Creator/1 -> alpha_chanel vars/1
  Sum/1 -> Bus Creator/3  "alpha_err"
  Ref Model and P Controller/3 -> Bus Creator/2, Sum/1  "alpha_sf"
  Ref Model and P Controller/2 -> Bus Creator/1  "alpha_sf_dot"
  Anti-windup AoA/1 -> Terminator2/1
  Anti-windup A_w_z/1 -> Terminator1/1
  A_w_z des/1 -> Terminator/1
  AoA des (rad)/1 -> Ref Model and P Controller/1
  Bus Selector/1 -> Ref Model and P Controller/2  "<AoA meas (rad)>"
  Ref Model and P Controller/1 -> alpha_dot_c/1
  All meas/1 -> Bus Selector/1

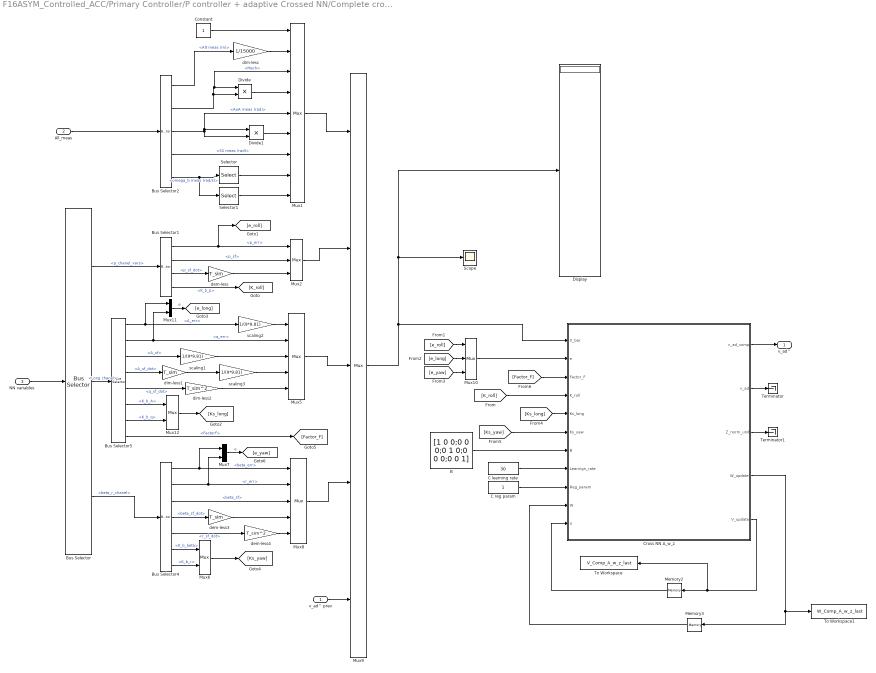
== system F16ASYM_Controlled_ACC/Primary Controller/P controller + adaptive Crossed NN/Complete crossed On-line (adaptive) multi-layer NN/Complete crossed On-line (adaptive) multi-layer NN: A_w_z ==
  v_ad^ prev : Inport
  All_meas : Inport  Port=2
  NN variables : Inport  Port=3
  B : Constant  Value=[1 0 0;0 0 0;0 1 0;0 0 0;0 0 1]
  Bus Selector : BusSelector  OutputSignals=p_chanel_vars,Long chanel,beta_r_chanel
  Bus Selector1 : BusSelector  OutputSignals=p_err,p_sf,p_sf_dot,K_b_p
  Bus Selector2 : BusSelector  OutputSignals=signal1.Alt meas (m),signal2.Mach,signal1.AoA meas (rad),signal1.SS meas (rad),signal1.omega_b meas (rad/s)
  Bus Selector4 : BusSelector  OutputSignals=beta_chanel vars.beta_err,r_chanel vars.r_err,beta_chanel vars.beta_sf,beta_chanel vars.beta_sf_dot,r_chanel vars.r_sf_dot,beta_chanel vars.K_b_beta,r_chanel vars.K_b_r
  Bus Selector5 : BusSelector  OutputSignals=A_chanel vars.A_err,q_chanel_vars.q_err,A_chanel vars.A_sf,A_chanel vars.A_sf_dot,q_chanel_vars.q_sf_dot,A_chanel vars.K_b_A,q_chanel_vars.K_b_q,A_chanel vars.FactorF
  C learning rate : Constant  Value=30  SampleTime=T_sim
  C reg param : Constant  SampleTime=T_sim
  Constant : Constant
  Cross NN A_w_z : MATLAB Function  TreatAsAtomicUnit=on
  Display : Display
  Divide : Product  Inputs=**
  Divide1 : Product  Inputs=**
  Memory2 : Memory  X0=V_Comp_A_w_z_last
  Memory3 : Memory  X0=W_Comp_A_w_z_last
  Mux1 : Mux  Inputs=9
  Mux10 : Mux  Inputs=3
  Mux{6..7,11..12} (4 alike) : Mux  Inputs=2
  Mux2 : Mux  Inputs=3
  Mux5 : Mux  Inputs=5
  Mux8 : Mux  Inputs=5
  Mux9 : Mux  Inputs=[9 3 5 5 3]
  Scope : Scope
      settings: SaveName=ScopeData8
  Selector : Selector  InputPortWidth=3  IndexOptions=Index vector (dialog)  Indices=1  OutputSizes=1
  Selector1 : Selector  InputPortWidth=3  IndexOptions=Index vector (dialog)  Indices=3  OutputSizes=1
  Terminator : Terminator
  Terminator1 : Terminator
  To Workspace : ToWorkspace  VariableName=V_Comp_A_w_z_last  SampleTime=-1
      settings: MaxDataPoints=1
  To Workspace1 : ToWorkspace  VariableName=W_Comp_A_w_z_last  SampleTime=-1
      settings: MaxDataPoints=1
  dem-less : Gain  Gain=T_sim
  dem-less3 : Gain  Gain=T_sim
  dem-less4 : Gain  Gain=T_sim^2
  dim-less : Gain  Gain=1/15000
  dim-less1 : Gain  Gain=T_sim
  dim-less2 : Gain  Gain=T_sim^2
  scaling1 : Gain  Gain=1/(9*9.81)
  scaling2 : Gain  Gain=1/(9*9.81)
  scaling3 : Gain  Gain=1/(9*9.81)
  v_ad^ : Outport
  wires:
  Bus Selector/3 -> Bus Selector4/1  "<beta_r_chanel>"
  Bus Selector/1 -> Bus Selector1/1  "<p_chanel_vars>"
  NN variables/1 -> Bus Selector/1
  Bus Selector2/5 -> Selector1/1, Selector/1  "<omega_b meas (rad/s)>"
  dim-less/1 -> Mux1/2
  Divide1/1 -> Mux1/6
  Divide/1 -> Mux1/4
  Bus Selector2/1 -> dim-less/1  "<Alt meas (m)>"
  All_meas/1 -> Bus Selector2/1
  Constant/1 -> Mux1/1
  Bus Selector1/3 -> dem-less/1  "<p_sf_dot>"
  Selector/1 -> Mux1/8
  Bus Selector2/4 -> Mux1/7  "<SS meas (rad)>"
  Bus Selector2/2 -> Divide/2, Mux1/3, Divide/1  "<Mach>"
  Bus Selector2/3 -> Divide1/1, Mux1/5, Divide1/2  "<AoA meas (rad)>"
  Bus Selector1/4 -> [K_roll]  "<K_b_p>"
  Bus Selector1/2 -> Mux2/2  "<p_sf>"
  Bus Selector1/1 -> [e_roll], Mux2/1  "<p_err>"
  dem-less/1 -> Mux2/3
  Mux12/1 -> [Ks_long]
  dem-less3/1 -> Mux8/4
  Bus Selector4/3 -> Mux8/3  "<beta_sf>"
  Bus Selector4/4 -> dem-less3/1  "<beta_sf_dot>"
  Bus Selector4/5 -> dem-less4/1  "<r_sf_dot>"
  Bus Selector4/7 -> Mux6/2  "<K_b_r>"
  Bus Selector4/6 -> Mux6/1  "<K_b_beta>"
  Mux6/1 -> [Ks_yaw]
  Bus Selector4/1 -> Mux8/1, Mux7/1  "<beta_err>"
  Bus Selector4/2 -> Mux8/2, Mux7/2  "<r_err>"
  Mux7/1 -> [e_yaw]  "e"
  dem-less4/1 -> Mux8/5
  Mux1/1 -> Mux9/1
  Mux2/1 -> Mux9/2
  Mux5/1 -> Mux9/3
  Mux8/1 -> Mux9/4
  v_ad^ prev/1 -> Mux9/5
  Mux9/1 -> Scope/1, Display/1, Cross NN A_w_z/1(X_bar)
  Cross NN A_w_z/3(Z_norm_unit) -> Terminator1/1
  C reg param/1 -> Cross NN A_w_z/9(Reg_param)
  C learning rate/1 -> Cross NN A_w_z/8(Learnign_rate)
  Cross NN A_w_z/1(v_ad_comp) -> v_ad^/1
  Memory2/1 -> Cross NN A_w_z/11(V)
  Memory3/1 -> Cross NN A_w_z/10(W)
  B/1 -> Cross NN A_w_z/7(B)
  Cross NN A_w_z/2(v_ad) -> Terminator/1
  Cross NN A_w_z/5(V_update) -> To Workspace/1, Memory2/1
  Cross NN A_w_z/4(W_update) -> Memory3/1, To Workspace1/1
  Mux10/1 -> Cross NN A_w_z/2(e)
  [e_roll] -> Mux10/1
  [e_long] -> Mux10/2
  [e_yaw] -> Mux10/3
  [K_roll] -> Cross NN A_w_z/4(K_roll)
  [Ks_long] -> Cross NN A_w_z/5(Ks_long)
  [Ks_yaw] -> Cross NN A_w_z/6(Ks_yaw)
  Selector1/1 -> Mux1/9
  dim-less1/1 -> scaling3/1
  scaling2/1 -> Mux5/1
  Bus Selector5/6 -> Mux12/1  "<K_b_A>"
  Bus Selector5/7 -> Mux12/2  "<K_b_q>"
  Bus Selector5/5 -> dim-less2/1  "<q_sf_dot>"
  Bus Selector5/4 -> dim-less1/1  "<A_sf_dot>"
  Bus Selector5/3 -> scaling1/1  "<A_sf>"
  Bus Selector5/2 -> Mux5/2, Mux11/2  "<q_err>"
  Bus Selector5/1 -> scaling2/1, Mux11/1  "<A_err>"
  Bus Selector/2 -> Bus Selector5/1  "<Long chanel>"
  Mux11/1 -> [e_long]  "e"
  scaling1/1 -> Mux5/3
  dim-less2/1 -> Mux5/5
  scaling3/1 -> Mux5/4
  Bus Selector5/8 -> [Factor_F]  "<FactorF>"
  [Factor_F] -> Cross NN A_w_z/3(Factor_F)

== system F16ASYM_Controlled_ACC/Primary Controller/P controller + adaptive Crossed NN/Complete crossed On-line (adaptive) multi-layer NN/Complete crossed On-line (adaptive) multi-layer NN: AoA ==
  v_ad^ prev : Inport
  All_meas : Inport  Port=2
  NN variables : Inport  Port=3
  B : Constant  Value=[1 0 0;0 0 0;0 1 0;0 0 0;0 0 1]
  Bus Selector : BusSelector  OutputSignals=p_chanel_vars,Long chanel,beta_r_chanel
  Bus Selector1 : BusSelector  OutputSignals=p_err,p_sf,p_sf_dot,K_b_p
  Bus Selector2 : BusSelector  OutputSignals=signal1.Alt meas (m),signal2.Mach,signal1.AoA meas (rad),signal1.SS meas (rad),signal1.omega_b meas (rad/s)
  Bus Selector3 : BusSelector  OutputSignals=alpha_chanel vars.alpha_err,q_chanel_vars.q_err,alpha_chanel vars.alpha_sf,alpha_chanel vars.alpha_sf_dot,q_chanel_vars.q_sf_dot,alpha_chanel vars.K_b_alpha,q_chanel_vars.K_b_q
  Bus Selector4 : BusSelector  OutputSignals=beta_chanel vars.beta_err,r_chanel vars.r_err,beta_chanel vars.beta_sf,beta_chanel vars.beta_sf_dot,r_chanel vars.r_sf_dot,beta_chanel vars.K_b_beta,r_chanel vars.K_b_r
  C Learning rate : Constant  Value=30  SampleTime=T_sim
  C Reg param : Constant  Value=0.5  SampleTime=T_sim
  Constant : Constant
  Cross NN : MATLAB Function  TreatAsAtomicUnit=on
  Display : Display
  Divide : Product  Inputs=**
  Divide1 : Product  Inputs=**
  Memory2 : Memory  X0=V_Comp_last
  Memory3 : Memory  X0=W_Comp_last
  Mux1 : Mux  Inputs=9
  Mux10 : Mux  Inputs=3
  Mux2 : Mux  Inputs=3
  Mux{3..4,6..7} (4 alike) : Mux  Inputs=2
  Mux5 : Mux  Inputs=5
  Mux8 : Mux  Inputs=5
  Mux9 : Mux  Inputs=[9 3 5 5 3]
  Scope : Scope
      settings: SaveName=ScopeData8
  Selector : Selector  InputPortWidth=3  IndexOptions=Index vector (dialog)  Indices=1  OutputSizes=1
  Selector1 : Selector  InputPortWidth=3  IndexOptions=Index vector (dialog)  Indices=3  OutputSizes=1
  Terminator : Terminator
  Terminator1 : Terminator
  To Workspace : ToWorkspace  VariableName=V_Comp_last  SampleTime=-1
      settings: MaxDataPoints=1
  To Workspace1 : ToWorkspace  VariableName=W_Comp_last  SampleTime=-1
      settings: MaxDataPoints=1
  dem-less : Gain  Gain=T_sim
  dem-less1 : Gain  Gain=T_sim
  dem-less2 : Gain  Gain=T_sim^2
  dem-less3 : Gain  Gain=T_sim
  dem-less4 : Gain  Gain=T_sim^2
  dim-less : Gain  Gain=1/15000
  v_ad^ : Outport
  wires:
  Selector1/1 -> Mux1/9
  [Ks_yaw] -> Cross NN/5(Ks_yaw)
  [Ks_long] -> Cross NN/4(Ks_long)
  [K_roll] -> Cross NN/3(K_roll)
  [e_yaw] -> Mux10/3
  [e_long] -> Mux10/2
  [e_roll] -> Mux10/1
  Mux10/1 -> Cross NN/2(e)
  Cross NN/4(W_update) -> To Workspace1/1, Memory3/1
  Cross NN/5(V_update) -> Memory2/1, To Workspace/1
  Cross NN/2(v_ad) -> Terminator/1
  B/1 -> Cross NN/6(B)
  Memory3/1 -> Cross NN/9(W)
  Memory2/1 -> Cross NN/10(V)
  Cross NN/1(v_ad_comp) -> v_ad^/1
  C Learning rate/1 -> Cross NN/7(Learnign_rate)
  C Reg param/1 -> Cross NN/8(Reg_param)
  Cross NN/3(Z_norm_unit) -> Terminator1/1
  Mux9/1 -> Cross NN/1(X_bar), Display/1, Scope/1
  v_ad^ prev/1 -> Mux9/5
  Mux8/1 -> Mux9/4
  Mux5/1 -> Mux9/3
  Mux2/1 -> Mux9/2
  Mux1/1 -> Mux9/1
  dem-less4/1 -> Mux8/5
  Mux7/1 -> [e_yaw]  "e"
  Bus Selector4/2 -> Mux7/2, Mux8/2  "<r_err>"
  Bus Selector4/1 -> Mux7/1, Mux8/1  "<beta_err>"
  Mux6/1 -> [Ks_yaw]
  Bus Selector4/6 -> Mux6/1  "<K_b_beta>"
  Bus Selector4/7 -> Mux6/2  "<K_b_r>"
  Bus Selector4/5 -> dem-less4/1  "<r_sf_dot>"
  Bus Selector4/4 -> dem-less3/1  "<beta_sf_dot>"
  Bus Selector4/3 -> Mux8/3  "<beta_sf>"
  dem-less3/1 -> Mux8/4
  Mux3/1 -> [e_long]  "e"
  Bus Selector3/3 -> Mux5/3  "<alpha_sf>"
  Bus Selector3/2 -> Mux3/2, Mux5/2  "<q_err>"
  Bus Selector3/1 -> Mux3/1, Mux5/1  "<alpha_err>"
  Bus Selector3/4 -> dem-less1/1  "<alpha_sf_dot>"
  Bus Selector3/5 -> dem-less2/1  "<q_sf_dot>"
  Bus Selector3/7 -> Mux4/2  "<K_b_q>"
  Bus Selector3/6 -> Mux4/1  "<K_b_alpha>"
  Mux4/1 -> [Ks_long]
  dem-less1/1 -> Mux5/4
  dem-less2/1 -> Mux5/5
  dem-less/1 -> Mux2/3
  Bus Selector1/1 -> Mux2/1, [e_roll]  "<p_err>"
  Bus Selector1/2 -> Mux2/2  "<p_sf>"
  Bus Selector1/4 -> [K_roll]  "<K_b_p>"
  Bus Selector2/3 -> Divide1/2, Mux1/5, Divide1/1  "<AoA meas (rad)>"
  Bus Selector2/2 -> Divide/1, Mux1/3, Divide/2  "<Mach>"
  Bus Selector2/4 -> Mux1/7  "<SS meas (rad)>"
  Selector/1 -> Mux1/8
  Bus Selector1/3 -> dem-less/1  "<p_sf_dot>"
  Constant/1 -> Mux1/1
  All_meas/1 -> Bus Selector2/1
  Bus Selector2/1 -> dim-less/1  "<Alt meas (m)>"
  Divide/1 -> Mux1/4
  Divide1/1 -> Mux1/6
  dim-less/1 -> Mux1/2
  Bus Selector2/5 -> Selector/1, Selector1/1  "<omega_b meas (rad/s)>"
  NN variables/1 -> Bus Selector/1
  Bus Selector/1 -> Bus Selector1/1  "<p_chanel_vars>"
  Bus Selector/2 -> Bus Selector3/1  "<Long chanel>"
  Bus Selector/3 -> Bus Selector4/1  "<beta_r_chanel>"

== matlab function F16ASYM_Controlled_ACC/Control allocator/Control allocator: RECONFIG/MATLAB Function ==
  data: Deflections input; Saturations output; Sup_lim input; Inf_lim input
function Saturations = Saturations(Deflections,Sup_lim,Inf_lim)
Saturations=zeros(7,1);

for i=1:7
    
    if Deflections(i)>=Sup_lim(i)
        Saturations(i)=1;
    elseif Deflections(i)<=Inf_lim(i)
        Saturations(i)=-1;
    else
        Saturations(i)=0;
    end
end

== matlab function F16ASYM_Controlled_ACC/Primary Controller/P controller + adaptive Crossed NN/Complete crossed On-line (adaptive) multi-layer NN/Complete crossed On-line (adaptive) multi-layer NN: A_w_z/Cross NN A_w_z ==
  data: X_bar input size=[25,1]; v_ad_comp output; e input; Factor_F input; K_roll input; Ks_long input; Ks_yaw input; B input; Learnign_rate input size=1; Reg_param input size=1; W input size=[3,51]; V input size=[50,25]; v_ad output; Z_norm_unit output; T_sim parameter; W_update output; V_update output
function [v_ad_comp,v_ad,Z_norm_unit,W_update,V_update]  = Cross_NN(X_bar,e,Factor_F, K_roll,Ks_long,Ks_yaw,B,Learnign_rate,Reg_param,W,V,T_sim)

%% Compute prelimiary parametes
% Compute P with regular Lyapunov equation solution
P_roll=1/K_roll;
P_long =  [   1/Ks_long(1) , Factor_F/(Ks_long(1)^2+Ks_long(1)*Ks_long(2));
     1/(Ks_long(1)^2+Ks_long(1)*Ks_long(2)) ,(Ks_long(1)^2+Ks_long(1)*Ks_long(2)+Factor_F^2)/(Ks_long(2)^2*Ks_long(1)+Ks_long(2)*Ks_long(1)^2) ];
P_yaw = [   1/Ks_yaw(1) , 1/(Ks_yaw(1)^2+Ks_yaw(1)*Ks_yaw(2));
     1/(Ks_yaw(1)^2+Ks_yaw(1)*Ks_yaw(2)) ,(Ks_yaw(1)^2+Ks_yaw(1)*Ks_yaw(2)+1)/(Ks_yaw(2)^2*Ks_yaw(1)+Ks_yaw(2)*Ks_yaw(1)^2) ];
 
P = blkdiag(P_roll,P_long,P_yaw);

% % % % Compute P with on-line Lyapunov equation solution
% % % CROSS = 0;
% % % A = [ -K_roll,0,CROSS,0,0;0,-Ks_long(1),1,0,0;
% % %     0,0,-Ks_long(2),0,0;0,0,0,-Ks_yaw(1),Factor_F;0,0,0,0,-Ks_yaw(2)];
% % % 
% % % coder.extrinsic('lyap')
% % % P = A;
% % % P = lyap(A,2*diag(ones(5,1)));



zeta= e'*P*B;

%% Feedforward
z = V*X_bar;
s=sigmoid(V*X_bar);

sigma = [1 ; s ];
% v_ad = W*sigma;

sigma_grad = (sigma.*(ones(size(sigma))-sigma));

%% Compute the gradients or adaptation laws
Gamma_w= Learnign_rate; % W learnign rate
Gamma_v= Learnign_rate; %V learning rate
lambda = Reg_param;

V_dot=zeros(size(V));
W_dot=zeros(size(W));

W_dot= -Gamma_w*(  (sigma - sigma_grad.*[1;z] )*zeta  )';
W_dot(:,2:end)= W_dot(:,2:end) - Gamma_w*lambda*norm(zeta)*(W(:,2:end));

M = W'*zeta'.*sigma_grad ;
V_dot= -Gamma_v*( M(2:end)*X_bar'  );
V_dot(:,2:end)= V_dot(:,2:end) - Gamma_v*lambda*norm(zeta).*V(:,2:end);

% % % % 
% % % % % Other way: Based on notes of Andrew NG
% % % % 
% % % % delta2=W'*zeta'.*sigma_grad;
% % % % 
% % % % V_dot = - Gamma_v*( delta2(2:end)*X_bar');
% % % % V_dot(:,2:end)= V_dot(:,2:end) - Gamma_v*lambda*norm(zeta).*V(:,2:end);
% % % % 
% % % % W_dot = - Gamma_w*( sigma*zeta)';
% % % % W_dot(:,2:end)= W_dot(:,2:end) - Gamma_w*lambda*norm(zeta)*(W(:,2:end));



%% Adaptation
W_update = W + T_sim*W_dot;
V_update = V + T_sim*V_dot;

%% Re-compute v_ad

s=sigmoid(V_update*X_bar);

sigma = [1 ; s(:,1) ];
v_ad = W_update*sigma;

%% Compute v_ad_comp
Z = [ V,zeros(size(V,1),size(W,2));
    zeros(size(W,1),size(V,2)),W];
    
Z_norm = norm(Z,'fro');
Z_max = 2*min(size(W,1),size(W,2) )*min( size(V,1),size(V,2) );
Z_norm_unit = Z_norm;

K_r0= 0.02;
K_r1= 0;
v_r0 = -K_r0*zeta';
v_r1 = -K_r1*(Z_norm+Z_max)*zeta';

v_ad_comp = v_ad + v_r1 +v_r0;


end

== matlab function F16ASYM_Controlled_ACC/Primary Controller/P controller + adaptive Crossed NN + AWU+Lim /Sigmoid /MATLAB Function ==
  data: u input; y output; a input
function y = sigmoid_a(u,a)

y = 2.0 ./ (1.0 + exp(-a*u(1:3)))-1;

== matlab function F16ASYM_Controlled_ACC/Primary Controller/P  + Crossed NN + AWU+Lim + hand-over/Transition smoother ==
  data: Comm output; AoA_comm input; indicator input; ACC_comm input; indicator_out output; indicator_prev input
function [Comm,indicator_out]  = Smoother(AoA_comm,indicator,ACC_comm,indicator_prev)

if indicator==indicator_prev
    indicator_out = indicator;
    if indicator==1
        Comm = AoA_comm;
    else
        Comm = ACC_comm;
    end
end

% Transition
